simulink model "full_task"  (R2025b)
settings: Solver=ode4  StartTime=0.0  StopTime=25.0  FixedStep=0.001  RelTol=1e-3
values from neighbouring files (symbols this model uses):
  K_posture = [100;100;0.01]    [posture_controllers.m]    (also in sim_FT.m = [10,10,100]; simulate_full_task.m = [10,10,100])
  KNL_b = 100    [sim_FT.m]    (also in simulate_configuration_control.m = 1; simulate_full_task.m; simulate_trajectory_tracking.m = 1; tracking_controllers.m = 1000)
  KNL_xi = 0.25    [sim_FT.m]    (also in simulate_configuration_control.m = 0.5; simulate_full_task.m; simulate_trajectory_tracking.m = 0.5; tracking_controllers.m = 0.9999)
  q0_dot_trajtrack = [-20; -4; 0]    [sim_FT.m]    (also in simulate_full_task.m)
  q0_posture = [err_mag;err_phase;delta_pos]    [posture_controllers.m]    (also in sim_FT.m = [rho_0; gamma_0; delta_0]; simulate_configuration_control.m; simulate_full_task.m = [rho_0; gamma_0; delta_0])
settings Model: Creator=matteo  LastModifiedBy=fede

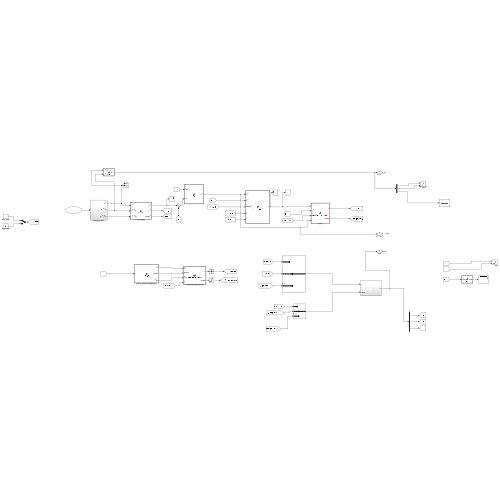
[thumbnail: Simulink's stored preview of the top-level diagram]
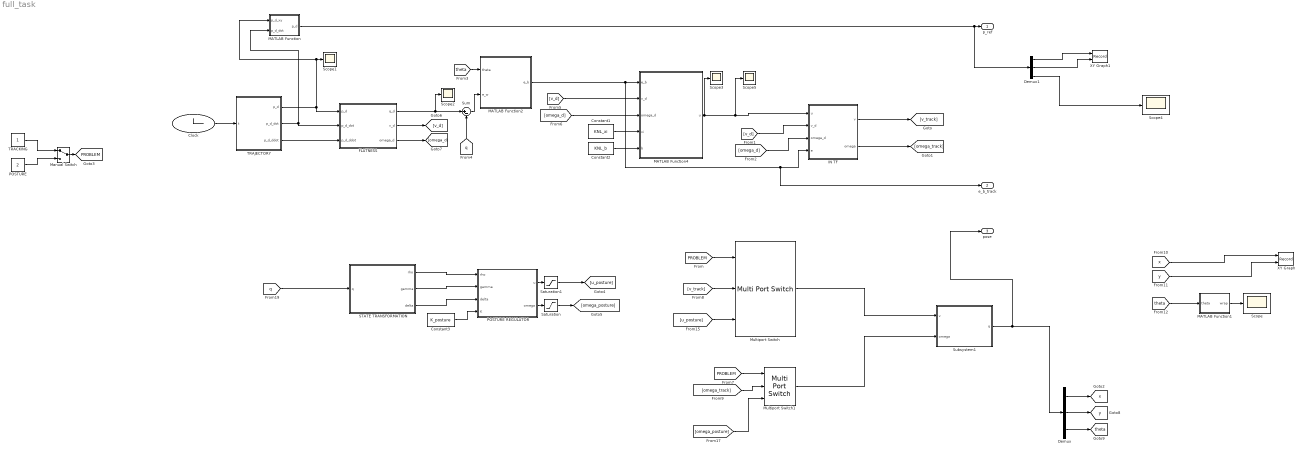
== system full_task ==
  Clock : Clock
      settings: Decimation=25
  Constant1 : Constant  Value=KNL_xi
  Constant2 : Constant  Value=KNL_b
  Constant3 : Constant  Value=K_posture
  Demux : Demux  Outputs=3
  Demux1 : Demux  Outputs=3
  FLATNESS : MATLAB Function  TreatAsAtomicUnit=on
  IN TF : MATLAB Function  TreatAsAtomicUnit=on
  MATLAB Function : MATLAB Function  TreatAsAtomicUnit=on
  MATLAB Function1 : MATLAB Function  TreatAsAtomicUnit=on
  MATLAB Function2 : MATLAB Function  TreatAsAtomicUnit=on
  MATLAB Function4 : MATLAB Function  TreatAsAtomicUnit=on
  Manual Switch : ManualSwitch
  Multiport Switch : MultiPortSwitch  Inputs=2  SaturateOnIntegerOverflow=off  InputSameDT=off
  Multiport Switch1 : MultiPortSwitch  Inputs=2  SaturateOnIntegerOverflow=off  InputSameDT=off
  POSTURE : Constant  Value=2
  POSTURE REGULATOR : MATLAB Function  TreatAsAtomicUnit=on
  STATE TRANSFORMATION : MATLAB Function  TreatAsAtomicUnit=on
  Saturation : Saturate  UpperLimit=100  LowerLimit=-100
  Saturation1 : Saturate  UpperLimit=5  LowerLimit=-5
  Scope{,1..5} (6 alike) : Scope
      Scope settings: ActiveDisplayYMinimum=-11.42914762924687  ActiveDisplayYMaximum=17.890956068905542
      Scope1 settings: ActiveDisplayYMinimum=-197.23068798329467  ActiveDisplayYMaximum=76.188437653574553
      Scope2 settings: ActiveDisplayYMinimum=-1  ActiveDisplayYMaximum=1  DataLoggingVariableName=ScopeData2
      Scope3 settings: ActiveDisplayYMinimum=-82.913496116494485  ActiveDisplayYMaximum=80.114760972742772  DataLoggingVariableName=ScopeData3
      Scope4 settings: ActiveDisplayYMinimum=-11.42914762924687  ActiveDisplayYMaximum=17.890956068905542  DataLoggingVariableName=ScopeData4
      Scope5 settings: ActiveDisplayYMinimum=-25.955730618951179  ActiveDisplayYMaximum=48.508278696051576  DataLoggingVariableName=ScopeData6
  Subsystem1 : Subsystem
  Sum : Sum  Inputs=|+-
  TRACKING : Constant
  TRAJECTORY : Subsystem
  XY Graph : Record  NumPorts=2.0  FileSettingsInternal="{\"entries\":[{\"content\":{\"excelSettings\":{\"content\":{},\"type\":\"Streamout.ExcelSettings\"},\"parquetSettings\":{\"content\":{},\"type\":\"Streamout.ParquetSettings\"}},\"type\":\"Streamout.FileSettingStorage\",\"uuid\":\"\"}],\"packageUris\":[\"http:\\/\\/schema.mathworks.com\\/mf0\\/streamout_blocks\\/R2020a\"],\"version\":\"1.0\"}"  FrameSettings=[0, 0]  Layout=[1 1]  SignalsInternal="{\"entries\":[{\"content\":{\"signals\":[{\"content\":{\"blockPath\":[],\"dimensions\":[1,1],\"domain\":\"\",\"lineColor\":\"#a2142f\",\"plots\":[ 1 ],\"port\":1,\"sid\":[\"\"],\"signalID\":1,\"signalName\":\"From10\"},\"type\":\"RecordBlkView.Signal\",\"uuid\":\"\"},{\"content\":{\"blockPath\":[],\"dimensions\":[1,1],\"domain\":\"\",\"lineColor\":\"#139fff\",\"plots\":[ 1 ],\"port\":2,\"sid\":[\"\"],\"signalID\":2,\"signalName\":\"From11\"},\"type\":\"RecordBlkView.Signal\",\"uuid\":\"\"}]},\"type\":\"RecordBlkView.InputSignals\",\"uuid\":\"\"}],\"packageUris\":[\"http:\\/\\/schema.mathworks.com\\/mf0\\/streamout_blocks\\/R2020a\"],\"version\":\"1.0\"}"  VisualizationBindings="{\"xyplotplugin\":{\"info\":[{\"series\":[{\"bindingParametersList\":[{\"parameter\":\"X-Axis\",\"signalID\":1,\"signalName\":\"From10\"},{\"parameter\":\"Y-Axis\",\"signalID\":2,\"signalName\":\"From11\"}],\"seriesID\":0}],\"subplotID\":1}]}}"  CompatibilityTag=XY
  XY Graph1 : Record  NumPorts=2.0  FileSettingsInternal="{\"entries\":[{\"content\":{\"excelSettings\":{\"content\":{},\"type\":\"Streamout.ExcelSettings\"},\"parquetSettings\":{\"content\":{},\"type\":\"Streamout.ParquetSettings\"}},\"type\":\"Streamout.FileSettingStorage\",\"uuid\":\"\"}],\"packageUris\":[\"http:\\/\\/schema.mathworks.com\\/mf0\\/streamout_blocks\\/R2020a\"],\"version\":\"1.0\"}"  FrameSettings=[0, 0]  Layout=[1 1]  SignalsInternal="{\"entries\":[{\"content\":{\"signals\":[{\"content\":{\"blockPath\":[],\"dimensions\":[1,1],\"domain\":\"\",\"lineColor\":\"#a2142f\",\"plots\":[ 1 ],\"port\":1,\"sid\":[\"\"],\"signalID\":1,\"signalName\":\"Demux1:1\"},\"type\":\"RecordBlkView.Signal\",\"uuid\":\"\"},{\"content\":{\"blockPath\":[],\"dimensions\":[1,1],\"domain\":\"\",\"lineColor\":\"#139fff\",\"plots\":[ 1 ],\"port\":2,\"sid\":[\"\"],\"signalID\":2,\"signalName\":\"Demux1:2\"},\"type\":\"RecordBlkView.Signal\",\"uuid\":\"\"}]},\"type\":\"RecordBlkView.InputSignals\",\"uuid\":\"\"}],\"packageUris\":[\"http:\\/\\/schema.mathworks.com\\/mf0\\/streamout_blocks\\/R2020a\"],\"version\":\"1.0\"}"  VisualizationBindings="{\"xyplotplugin\":{\"info\":[{\"series\":[{\"bindingParametersList\":[{\"parameter\":\"X-Axis\",\"signalID\":1,\"signalName\":\"Demux1:1\"},{\"parameter\":\"Y-Axis\",\"signalID\":2,\"signalName\":\"Demux1:2\"}],\"seriesID\":0}],\"subplotID\":1}]}}"  CompatibilityTag=XY
  p_ref : Outport  SignalName=p_ref
  e_b_track : Outport  Port=2  SignalName=e_b_track
  pose : Outport  Port=3  SignalName=pose
  tag scope: PROBLEM=global, theta=global, x=global, y=global
  wires:
  TRACKING/1 -> Manual Switch/1
  Manual Switch/1 -> [PROBLEM]
  POSTURE/1 -> Manual Switch/2
  Clock/1 -> TRAJECTORY/1(t)
  TRAJECTORY/1(p_d) -> FLATNESS/1(p_d), MATLAB Function/1(p_d_xy), Scope1/1
  MATLAB Function/1(p_d) -> Demux1/1, p_ref/1
  TRAJECTORY/2(p_d_dot) -> FLATNESS/2(p_d_dot), MATLAB Function/2(p_d_dot)
  TRAJECTORY/3(p_d_ddot) -> FLATNESS/3(p_d_ddot)
  FLATNESS/2(v_d) -> [v_d]
  FLATNESS/3(omega_d) -> [omega_d]
  Sum/1 -> MATLAB Function2/2(e_w)
  FLATNESS/1(q_d) -> Scope2/1, Sum/1
  [theta] -> MATLAB Function2/1(theta)
  [q] -> Sum/2
  [omega_d] -> MATLAB Function4/3(omega_d)
  Constant2/1 -> MATLAB Function4/5(b)
  MATLAB Function2/1(e_b) -> MATLAB Function4/1(e_b), e_b_track/1, IN TF/4(e)
  Constant1/1 -> MATLAB Function4/4(xi)
  [v_d] -> MATLAB Function4/2(v_d)
  [v_d] -> IN TF/2(v_d)
  [omega_d] -> IN TF/3(omega_d)
  IN TF/1(v) -> [v_track]
  IN TF/2(omega) -> [omega_track]
  POSTURE REGULATOR/1(u) -> Saturation1/1
  Constant3/1 -> POSTURE REGULATOR/4(K)
  [q] -> STATE TRANSFORMATION/1(q)
  STATE TRANSFORMATION/1(rho) -> POSTURE REGULATOR/1(rho)
  STATE TRANSFORMATION/2(gamma) -> POSTURE REGULATOR/2(gamma)
  STATE TRANSFORMATION/3(delta) -> POSTURE REGULATOR/3(delta)
  [PROBLEM] -> Multiport Switch1/1
  [omega_track] -> Multiport Switch1/2
  [PROBLEM] -> Multiport Switch/1
  [omega_posture] -> Multiport Switch1/3
  [u_posture] -> Multiport Switch/3
  [v_track] -> Multiport Switch/2
  Demux/2 -> [y]
  Multiport Switch1/1 -> Subsystem1/2(omega)
  Multiport Switch/1 -> Subsystem1/1(v)
  Demux/3 -> [theta]
  Demux/1 -> [x]
  Subsystem1/1(q) -> Demux/1, pose/1
  [theta] -> MATLAB Function1/1(theta)
  MATLAB Function1/1(wrap) -> Scope/1
  Demux1/3 -> Scope4/1
  [x] -> XY Graph/1
  [y] -> XY Graph/2
  Demux1/1 -> XY Graph1/1
  Demux1/2 -> XY Graph1/2
  MATLAB Function4/1(u) -> Scope5/1, IN TF/1(u), Scope3/1
  POSTURE REGULATOR/2(omega) -> Saturation/1
  Saturation/1 -> [omega_posture]
  Saturation1/1 -> [u_posture]

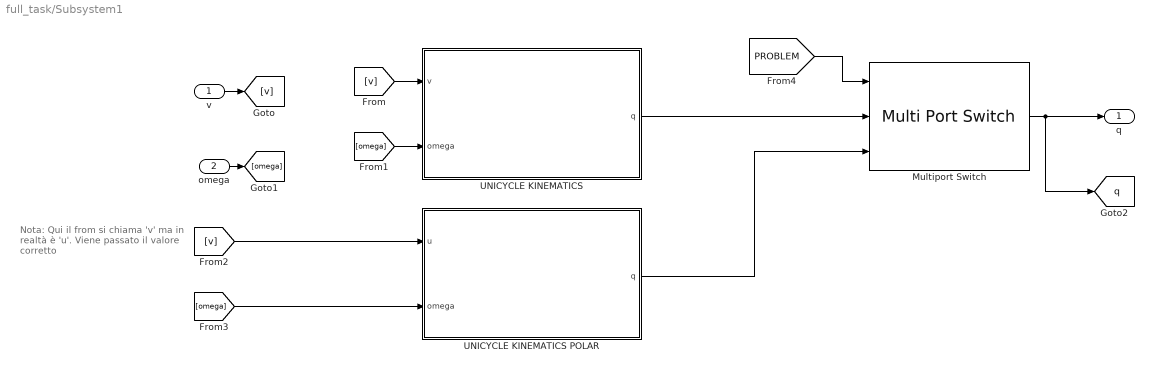
== system full_task/Subsystem1 ==
  note: Nota: Qui il from si chiama 'v' ma in
      | realtà è 'u'. Viene passato il valore
      | corretto
  v : Inport
  omega : Inport  Port=2
  Multiport Switch : MultiPortSwitch  Inputs=2  SaturateOnIntegerOverflow=off  InputSameDT=off
  UNICYCLE KINEMATICS : Subsystem
  UNICYCLE KINEMATICS POLAR : Subsystem
  q : Outport
  tag scope: q=global
  wires:
  Multiport Switch/1 -> [q], q/1
  UNICYCLE KINEMATICS/1(q) -> Multiport Switch/2
  v/1 -> [v]
  omega/1 -> [omega]
  [omega] -> UNICYCLE KINEMATICS/2(omega)
  [v] -> UNICYCLE KINEMATICS/1(v)
  [v] -> UNICYCLE KINEMATICS POLAR/1(u)
  [omega] -> UNICYCLE KINEMATICS POLAR/2(omega)
  [PROBLEM] -> Multiport Switch/1
  UNICYCLE KINEMATICS POLAR/1(q) -> Multiport Switch/3

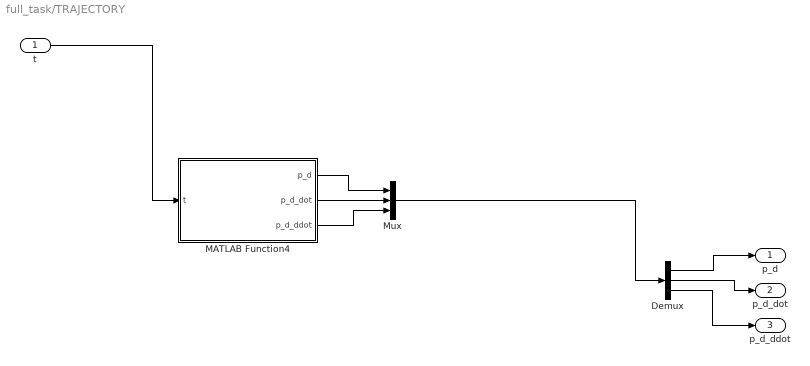
== system full_task/TRAJECTORY ==
  t : Inport
  Demux : Demux  Outputs=3
  MATLAB Function4 : MATLAB Function  TreatAsAtomicUnit=on
  Mux : Mux  Inputs=3
  p_d : Outport
  p_d_dot : Outport  Port=2
  p_d_ddot : Outport  Port=3
  wires:
  t/1 -> MATLAB Function4/1(t)
  MATLAB Function4/1(p_d) -> Mux/1
  MATLAB Function4/2(p_d_dot) -> Mux/2
  MATLAB Function4/3(p_d_ddot) -> Mux/3
  Mux/1 -> Demux/1
  Demux/1 -> p_d/1
  Demux/2 -> p_d_dot/1
  Demux/3 -> p_d_ddot/1

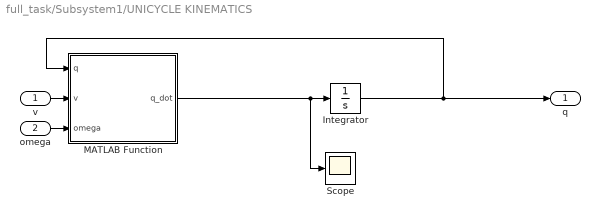
== system full_task/Subsystem1/UNICYCLE KINEMATICS ==
  v : Inport
  omega : Inport  Port=2
  Integrator : Integrator  InitialCondition=q0_dot_trajtrack
  MATLAB Function : MATLAB Function  TreatAsAtomicUnit=on
  Scope : Scope
      settings: ActiveDisplayYMinimum=-172.45764513184179  ActiveDisplayYMaximum=196.48761534542967  DataLoggingVariableName=ScopeData5
  q : Outport
  wires:
  v/1 -> MATLAB Function/2(v)
  omega/1 -> MATLAB Function/3(omega)
  Integrator/1 -> q/1, MATLAB Function/1(q)
  MATLAB Function/1(q_dot) -> Scope/1, Integrator/1

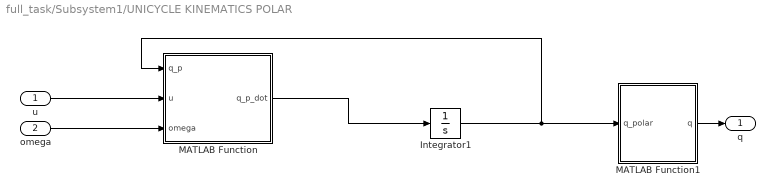
== system full_task/Subsystem1/UNICYCLE KINEMATICS POLAR ==
  u : Inport
  omega : Inport  Port=2
  Integrator1 : Integrator  InitialCondition=q0_posture
  MATLAB Function : MATLAB Function  TreatAsAtomicUnit=on
  MATLAB Function1 : MATLAB Function  TreatAsAtomicUnit=on
  q : Outport
  wires:
  u/1 -> MATLAB Function/2(u)
  omega/1 -> MATLAB Function/3(omega)
  Integrator1/1 -> MATLAB Function1/1(q_polar), MATLAB Function/1(q_p)
  MATLAB Function1/1(q) -> q/1
  MATLAB Function/1(q_p_dot) -> Integrator1/1

== matlab function full_task/STATE TRANSFORMATION ==
  data: rho output; q input; gamma output; delta output
function [rho, gamma, delta] = state_tf(q)


x = q(1);
y = q(2);
theta = q(3);

rho = sqrt(x^2+y^2);
gamma = atan2(y,x)+pi-theta;
delta = gamma+theta;

== matlab function full_task/Subsystem1/UNICYCLE KINEMATICS POLAR/MATLAB Function1 ==
  data: q_polar input; q output
function q = inv_state_tf(q_polar)

rho = q_polar(1);
gamma = q_polar(2);
delta = q_polar(3);


x = -rho*cos(delta);
y = -rho*sin(delta);
theta = delta - gamma;

q = [x; y; theta];

== matlab function full_task/Subsystem1/UNICYCLE KINEMATICS/MATLAB Function ==
  data: q input; q_dot output; v input; omega input
function q_dot = fcn(q, v, omega)
%write the unicycle model
q_dot= zeros(3,1);

q_dot(1) = v*cos(q(3));
q_dot(2) = v*sin(q(3));
q_dot(3) = omega;

== matlab function full_task/MATLAB Function1 ==
  data: theta input; wrap output
function wrap = fcn(theta)

wrap = mod(theta+pi,2*pi)-pi ;

== matlab function full_task/MATLAB Function2 ==
  data: theta input; e_b output; e_w input
function e_b = Rz(theta, e_w)

e_b = zeros(3,1);
e_b(1)=cos(theta)*e_w(1)+sin(theta)*e_w(2);
e_b(2)=-sin(theta)*e_w(1)+cos(theta)*e_w(2);
e_b(3)=e_w(3);

== matlab function full_task/IN TF ==
  data: u input; v output; omega output; v_d input; omega_d input; e input
function [v, omega] = input_transformation(u, v_d, omega_d,e)
v= 0;
omega = 0;
v = v_d*cos(e(3))-u(1);
omega = omega_d-u(2);

== matlab function full_task/MATLAB Function4 ==
  data: e_b input; u output; v_d input; omega_d input size=1; xi input size=1; b input size=1
function u = nonlinear_gain(e_b, v_d, omega_d, xi, b)

K2 = b;
K1 = 2*xi*sqrt(b*v_d+omega_d^2);
K3 = 2*xi*sqrt(b*v_d+omega_d^2);

u=zeros(2,1);
u(1) = -K1*e_b(1);
u(2) = -K2*v_d*e_b(2)*sin(e_b(3))/(sign(e_b(3))*sqrt((e_b(3)+1e-6)^2))-K3*e_b(3);

% Angular velocity command (with singularity protection)
% Use a threshold to avoid division by zero
if abs(e_b(3)) < 1e-5
    % Limit: sin(x)/x as x -> 0 is 1
    sinc = 1.0;
else
    sinc = sin(e_b(3)) / e_b(3);
end

% u(2) = -K2 * v_d * e_b(2) * [sin(e_theta)/e_theta] - K3 * e_theta
u(2) = -K2 * v_d * e_b(2) * sinc - K3 * e_b(3);

== matlab function full_task/FLATNESS ==
  data: p_d input; q_d output; v_d output; omega_d output; p_d_dot input; p_d_ddot input
function [q_d, v_d, omega_d] = flatness(p_d, p_d_dot, p_d_ddot)

x = p_d(1);
y = p_d(2);

x_dot = p_d_dot(1);
y_dot = p_d_dot(2);

x_ddot = p_d_ddot(1);
y_ddot = p_d_ddot(2);

% velocità
v_d = sqrt(x_dot^2 + y_dot^2);

% orientamento
theta_d = atan2(y_dot, x_dot);

% velocità angolare
den = x_dot^2 + y_dot^2;

if den < 1e-8
    omega_d = 0;
else
    omega_d = (x_dot*y_ddot - y_dot*x_ddot)/den;
end

% stato desiderato
q_d = [x; y; theta_d];

end

== matlab function full_task/TRAJECTORY/MATLAB Function4 ==
  data: t input; p_d output; p_d_dot output; p_d_ddot output
function [p_d, p_d_dot, p_d_ddot] = parking_trajectory(t)
    % Total time: 25s (5s per segment)
    % Segments: 
    % 1: Rect (Start -> -16, -2)
    % 2: Ellipse (-16, -2 -> -10, -8) [Bending Down]
    % 3: Circle/Ellipse (-10, -8 -> -7, -14 -> -4, -8) [Bending Down]
    % 4: Zigzag (-4, -8 -> -4, -4) [Moving Up]
    % 5: Rect (-4, -4 -> -4, -2 -> 0, -2)
    
    if t < 5
        %% SEGMENT 1: RECTANGULAR
        % Path: (-20, -4) -> (-20, -2) [Up] -> (-16, -2) [Right]
        t_rel = t;
        T_side = 2.5; 
        v_v = 0.8; v_h = 1.6; 
        
        if t_rel < T_side
            p_d = [-20; -4 + v_v*t_rel];
            p_d_dot = [0; v_v];
        else
            p_d = [-20 + v_h*(t_rel-T_side); -2];
            p_d_dot = [v_h; 0];
        end
        p_d_ddot = [0; 0];

    elseif t < 10
        %% SEGMENT 2: ELLIPTICAL (Bending Downwards)
        % Start: (-16, -2), End: (-10, -8)
        % Center: (-16, -8), a=6, b=6
        t_rel = t - 5;
        omega = (pi/2) / 5; 
        a = 6; b = 6;
        xc = -16; yc = -8;
        
        % Angle goes from pi/2 down to 0
        theta = pi/2 - omega*t_rel;
        
        p_d = [xc + a*cos(theta); yc + b*sin(theta)];
        p_d_dot = [-a*omega*sin(theta); -b*omega*cos(theta)];
        p_d_ddot = [-a*omega^2*cos(theta); -b*omega^2*sin(theta)];

    elseif t < 15
        %% SEGMENT 3: CIRCULAR (Valley Shape)
        % Start: (-10, -8), Apex: (-7, -11), End: (-4, -8)
        % Center: (-7, -8), a=3, b=3
        t_rel = t - 10;
        omega = pi / 5; 
        a = 3; b = 3;
        xc = -7; yc = -8;
        
        % Angle goes from pi to 2*pi
        theta = pi + omega*t_rel;
        
        p_d = [xc + a*cos(theta); yc + b*sin(theta)];
        p_d_dot = [-a*omega*sin(theta); b*omega*cos(theta)];
        p_d_ddot = [-a*omega^2*cos(theta); -b*omega^2*sin(theta)];

    elseif t < 20
        %% SEGMENT 4: ZIGZAG (Moving Upwards)
        % Moving from (-4, -8) up to (-4, -4)
        t_rel = t - 15;
        A = 1.5;              
        T_zz = 2.5;      
        v_y = 0.8; % Speed: ((-4) - (-8)) / 5s = 0.8 m/s
        vy_speed = (4 * A) / T_zz; 
        
        y = -8 + v_y * t_rel;
        t_osc = mod(t_rel, T_zz);
        if t_osc < T_zz/4
            x = -4 + vy_speed * t_osc;
            vx = vy_speed;
        elseif t_osc < 3*T_zz/4
            x = -4 + A - vy_speed * (t_osc - T_zz/4);
            vx = -vy_speed;
        else
            x = -4 - A + vy_speed * (t_osc - 3*T_zz/4);
            vx = vy_speed;
        end
        p_d = [x; y];
        p_d_dot = [vx; v_y];
        p_d_ddot = [0; 0];

    else
        %% SEGMENT 5: RECTANGULAR
        % Vertical part: 20s to 22.5s (Path: (-4, -4) -> (-4, -2))
        % Horizontal part: 22.5s to 25s (Path: (-4, -2) -> (0, -2))
        t_rel = t - 20;
        T_side = 2.5;
        
        if t_rel < T_side
            % --- VERTICAL PART (Moving Up) ---
            v_v = 0.8; % Speed: ((-2) - (-4)) / 2.5s = 0.8 m/s
            p_d = [-4; -4 + v_v * t_rel];
            p_d_dot = [0; v_v];
            p_d_ddot = [0; 0];
        else
            % --- HORIZONTAL PART (Deceleration to v=0.25) ---
            t_h = t_rel - T_side;
            
            % Kinematic Parameters (Distance = 4m, Time = 2.5s)
            v0 = 2.95;
            a_accel = -1.08;
            
            vx = v0 + a_accel * t_h;
            x = -4 + v0 * t_h + 0.5 * a_accel * t_h^2;
            
            p_d = [x; -2];
            p_d_dot = [vx; 0];
            p_d_ddot = [a_accel; 0]; 
        end
    end
end

== matlab function full_task/MATLAB Function ==
  data: p_d_xy input; p_d output; p_d_dot input
function p_d = fcn(p_d_xy, p_d_dot)
    x = p_d_xy(1);
    y = p_d_xy(2);
    
    vx = p_d_dot(1);
    vy = p_d_dot(2);
    
    % Heading is the angle of the velocity vector
    theta = atan2(vy, vx); 
    
    p_d = [x; y; theta];
end

== matlab function full_task/Subsystem1/UNICYCLE KINEMATICS POLAR/MATLAB Function ==
  data: q_p input; q_p_dot output; u input; omega input
function q_p_dot = fcn(q_p, u, omega)
%write the unicycle model
q_p_dot= zeros(3,1);
rho = q_p(1);
gamma = q_p(2);

q_p_dot(1) = -u*cos(gamma);
q_p_dot(2) = sin(gamma)*u-omega;
q_p_dot(3) = sin(gamma)*u;

== matlab function full_task/POSTURE REGULATOR ==
  data: u output; omega output; rho input; gamma input; delta input; K input
function [u, omega] = posture_regulator(rho, gamma, delta, K)

u = K(1)*rho*cos(gamma);
%u = K(1)*cos(gamma);
omega = K(2)*gamma + K(1)*((sin(gamma)*cos(gamma))/gamma) *(gamma+K(3)*delta);
